simulink model "Tethered_Wind_Tunnel_Test"  (R2023a)
settings: Solver=VariableStepAuto  StartTime=0.0  StopTime=10.0  RelTol=1e-3
values from neighbouring files (symbols this model uses):
  b = 0.490    (= 0.49)    [Cascaded_PI_Step.m]    (also in Cascaded_PI_Zero_Ref.m; Gain_Scheduled_PI_Step.m; Gain_Scheduled_PI_Zero_Ref.m; Inner_Loop_Relay_Feedback.m)
  Bc = 0    [Tethered_Wind_Tunnel.m]
  c = 0.0885    [Tethered_Wind_Tunnel.m]
  Clbc = 1    [Tethered_Wind_Tunnel.m]
  Clda = 0.65    [Cascaded_PI_Step.m]    (also in Cascaded_PI_Zero_Ref.m; Gain_Scheduled_PI_Step.m; Gain_Scheduled_PI_Zero_Ref.m; Inner_Loop_Relay_Feedback.m)
  Cldr = -0.005    [Tethered_Wind_Tunnel.m]
  Clo = 1.108    [Cascaded_PI_Step.m]    (also in Cascaded_PI_Zero_Ref.m; Gain_Scheduled_PI_Step.m; Gain_Scheduled_PI_Zero_Ref.m; Inner_Loop_Relay_Feedback.m)
  Clp = -1.5    [Cascaded_PI_Step.m]    (also in Cascaded_PI_Zero_Ref.m = -11.5; Gain_Scheduled_PI_Step.m = -11.5; Gain_Scheduled_PI_Zero_Ref.m = -11.5; Inner_Loop_Relay_Feedback.m = -11.5)
  Clr = -15.4    [Tethered_Wind_Tunnel.m]
  Cma = -1.26    [Tethered_Wind_Tunnel.m]
  Cmde = 1.34    [Tethered_Wind_Tunnel.m]
  Cmo = 1    [Tethered_Wind_Tunnel.m]
  Cmq = -20.8    [Tethered_Wind_Tunnel.m]
  Cnbc = 1    [Tethered_Wind_Tunnel.m]
  Cnda = -0.065    [Tethered_Wind_Tunnel.m]
  Cndr = 0.005    [Tethered_Wind_Tunnel.m]
  Cno = 1.108    [Tethered_Wind_Tunnel.m]
  Cnp = -12    [Tethered_Wind_Tunnel.m]
  Cnr = -15    [Tethered_Wind_Tunnel.m]
  Gamma1 = (Ixz*(Ix-Iy-Iz))/Gamma0    (= 17.8020633247)    [Tethered_Wind_Tunnel.m]
  Gamma2 = (Iz*(Iz-Iy)+(Ixz^2))/Gamma0    (= -16.6988378289)    [Tethered_Wind_Tunnel.m]
  Gamma5 = (Iz-Ix)/Iy    (= 0.315753887762)    [Tethered_Wind_Tunnel.m]
  Gamma6 = Ixz/Gamma0    (= -13.0686120428)    [Tethered_Wind_Tunnel.m]
  Gamma7 = ((Ix-Iy)*Ix+Ixz^2)/Gamma0    (= -12.4708347919)    [Tethered_Wind_Tunnel.m]
  Iy = 1.0353    [Tethered_Wind_Tunnel.m]
  Kc2 = 7.67    [Cascaded_PI_Step.m]    (also in Cascaded_PI_Zero_Ref.m; Gain_Scheduled_PI_Step.m; Gain_Scheduled_PI_Zero_Ref.m; Tethered_Wind_Tunnel.m)
  Kc3 = 4.5    [Tethered_Wind_Tunnel.m]
  Kc4 = 0.87    [Tethered_Wind_Tunnel.m]
  Kc5 = 0.55    [Tethered_Wind_Tunnel.m]
  phi_des = 30    [Cascaded_PI_Step.m]    (also in Cascaded_PI_Zero_Ref.m = 0; Gain_Scheduled_PI_Step.m; Gain_Scheduled_PI_Zero_Ref.m = 0; Outer_Loop_Relay_Feedback.m = 20)
  r_des = 1    [Tethered_Wind_Tunnel.m]
  rho = 1.204    [Cascaded_PI_Step.m]    (also in Cascaded_PI_Zero_Ref.m; Gain_Scheduled_PI_Step.m; Gain_Scheduled_PI_Zero_Ref.m; Inner_Loop_Relay_Feedback.m)
  S = 0.44    [Cascaded_PI_Step.m]    (also in Cascaded_PI_Zero_Ref.m; Gain_Scheduled_PI_Step.m; Gain_Scheduled_PI_Zero_Ref.m; Inner_Loop_Relay_Feedback.m)
  tau2 = 24.12    [Cascaded_PI_Step.m]    (also in Cascaded_PI_Zero_Ref.m; Gain_Scheduled_PI_Step.m; Gain_Scheduled_PI_Zero_Ref.m; Tethered_Wind_Tunnel.m)
  tau3 = 20.12    [Tethered_Wind_Tunnel.m]
  tau4 = 0.10    (= 0.1)    [Tethered_Wind_Tunnel.m]
  tau5 = 1.25    [Tethered_Wind_Tunnel.m]
  theta_des = 7    [Tethered_Wind_Tunnel.m]
  Va = 15    [Cascaded_PI_Step.m]    (also in Cascaded_PI_Zero_Ref.m; Gain_Scheduled_PI_Step.m; Gain_Scheduled_PI_Zero_Ref.m; Inner_Loop_Relay_Feedback.m)
libraries: slpidlib x5
settings Model: Creator=brend  LastModifiedBy=brend

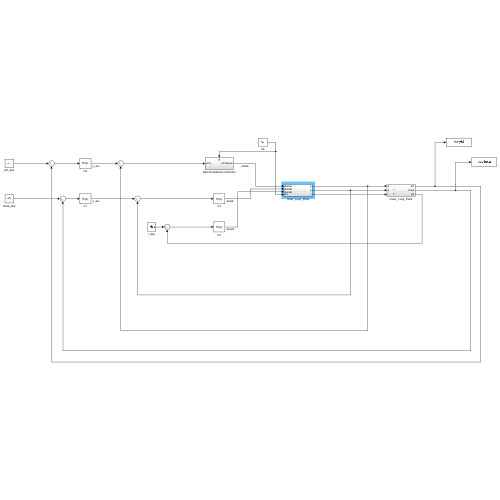
[thumbnail: Simulink's stored preview of the top-level diagram]
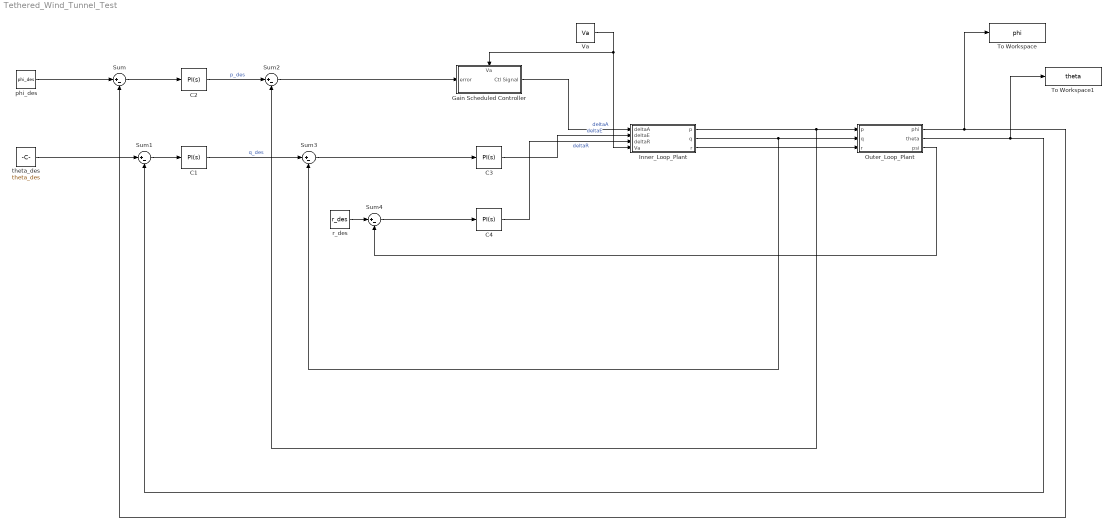
== system Tethered_Wind_Tunnel_Test ==
  C1 : slpidlib/PID Controller  Controller=PI  Form=Parallel  TimeDomain=Continuous-time  UseExternalTs=off  SampleTime=-1  IntegratorMethod=Forward Euler  FilterMethod=Forward Euler  ControllerParametersSource=internal  P=Kc3  I=tau3  UseKiTs=off  D=0  N=100  UseFilter=on  TunerSelectOption=Transfer Function Based (PID Tuner App)  InitialConditionSource=internal  InitialConditionForIntegrator=0  InitialConditionForFilter=0  DifferentiatorICPrevScaledInput=0  ExternalReset=none  TrackingMode=off  Kt=1  LimitOutput=off  SatLimitsSource=internal  UpperSaturationLimit=inf  LowerSaturationLimit=-inf  LinearizeAsGain=on  AntiWindupMode=none  Kb=1  LimitIntegrator=off  UpperIntegratorSaturationLimit=inf  LowerIntegratorSaturationLimit=-inf  POutMin=[]  POutMax=[]  IOutMin=[]  IOutMax=[]  DOutMin=[]  DOutMax=[]  NOutMin=[]  NOutMax=[]  SumOutMin=[]  SumOutMax=[]  SaturationOutMin=[]  SaturationOutMax=[]  PParamMin=[]  PParamMax=[]  IParamMin=[]  IParamMax=[]  DParamMin=[]  DParamMax=[]  NParamMin=[]  NParamMax=[]  KbParamMin=[]  KbParamMax=[]  KtParamMin=[]  KtParamMax=[]  KbOutMin=[]  KbOutMax=[]  KtOutMin=[]  KtOutMax=[]  IntegratorOutMin=[]  IntegratorOutMax=[]  FilterOutMin=[]  FilterOutMax=[]  SumI1OutMin=[]  SumI1OutMax=[]  SumI2OutMin=[]  SumI2OutMax=[]  SumI3OutMin=[]  SumI3OutMax=[]  SumI4OutMin=[]  SumI4OutMax=[]  SumDOutMin=[]  SumDOutMax=[]  DifferentiatorOutMin=[]  DifferentiatorOutMax=[]  FilterDiffOutCoefMin=[]  FilterDiffOutCoefMax=[]  ReciprocalOutMin=[]  ReciprocalOutMax=[]  SumDenOutMin=[]  SumDenOutMax=[]  SumNumOutMin=[]  SumNumOutMax=[]  DivideOutMin=[]  DivideOutMax=[]  UdiffTsProdOutMin=[]  UdiffTsProdOutMax=[]  NTsProdOutMin=[]  NTsProdOutMax=[]  UintegralTsProdOutMin=[]  UintegralTsProdOutMax=[]  UngainTsProdOutMin=[]  UngainTsProdOutMax=[]  ClampingZeroOutDataTypeStr=Inherit: Inherit via back propagation  ClampingZeroOutMin=[]  ClampingZeroOutMax=[]  FilterDenConstantOutDataTypeStr=Inherit: Inherit via back propagation  FilterDenConstantOutMin=[]  FilterDenConstantOutMax=[]  PCopyOutDataTypeStr=Inherit: Inherit via back propagation  PCopyOutMin=[]  PCopyOutMax=[]  NCopyOutDataTypeStr=Inherit: Inherit via back propagation  NCopyOutMin=[]  NCopyOutMax=[]  IntegratorContinuousStateAttributes=''  IntegratorStateMustResolveToSignalObject=off  IntegratorRTWStateStorageClass=Auto  FilterContinuousStateAttributes=''  FilterStateMustResolveToSignalObject=off  FilterRTWStateStorageClass=Auto  ParallelPVariant=InternalParameters  IdealPVariant=Disabled  IVariant=InternalParameters  DVariant=Disabled  IntegratorVariant=Continuous  SatVariant=Disabled  AWVariant=Passthrough  PCopyVariant=Disabled  TRVariant=Disabled  FdbkBlocksVariant=Forward  IdealPFdbkVariant=Disabled  SatFdbkVariant=Disabled  DerivativeFilterVariant=Disabled  NVariant=Disabled  NCopyVariant=Disabled_SignalSpec  FilterICVariant=Disabled  IntegratorICVariant=InternalICs  ExternalResetVariant=Disabled  TRSumVariant=Passthrough  SumFdbkVariant=Disabled  SumVariant=Sum_PI  TsampFilterVariant=InternalTs  TsampNgainVariant=Passthrough  TsampIntegralVariant=Disabled_SignalSpec  ExternalSaturationOutDataTypeStr=Inherit: Same as second input
  C2 : slpidlib/PID Controller  Controller=PI  Form=Parallel  TimeDomain=Continuous-time  UseExternalTs=off  SampleTime=-1  IntegratorMethod=Forward Euler  FilterMethod=Forward Euler  ControllerParametersSource=internal  P=Kc2  I=tau2  UseKiTs=off  D=0  N=100  UseFilter=on  TunerSelectOption=Transfer Function Based (PID Tuner App)  InitialConditionSource=internal  InitialConditionForIntegrator=0  InitialConditionForFilter=0  DifferentiatorICPrevScaledInput=0  ExternalReset=none  TrackingMode=off  Kt=1  LimitOutput=off  SatLimitsSource=internal  UpperSaturationLimit=inf  LowerSaturationLimit=-inf  LinearizeAsGain=on  AntiWindupMode=none  Kb=1  LimitIntegrator=off  UpperIntegratorSaturationLimit=inf  LowerIntegratorSaturationLimit=-inf  POutMin=[]  POutMax=[]  IOutMin=[]  IOutMax=[]  DOutMin=[]  DOutMax=[]  NOutMin=[]  NOutMax=[]  SumOutMin=[]  SumOutMax=[]  SaturationOutMin=[]  SaturationOutMax=[]  PParamMin=[]  PParamMax=[]  IParamMin=[]  IParamMax=[]  DParamMin=[]  DParamMax=[]  NParamMin=[]  NParamMax=[]  KbParamMin=[]  KbParamMax=[]  KtParamMin=[]  KtParamMax=[]  KbOutMin=[]  KbOutMax=[]  KtOutMin=[]  KtOutMax=[]  IntegratorOutMin=[]  IntegratorOutMax=[]  FilterOutMin=[]  FilterOutMax=[]  SumI1OutMin=[]  SumI1OutMax=[]  SumI2OutMin=[]  SumI2OutMax=[]  SumI3OutMin=[]  SumI3OutMax=[]  SumI4OutMin=[]  SumI4OutMax=[]  SumDOutMin=[]  SumDOutMax=[]  DifferentiatorOutMin=[]  DifferentiatorOutMax=[]  FilterDiffOutCoefMin=[]  FilterDiffOutCoefMax=[]  ReciprocalOutMin=[]  ReciprocalOutMax=[]  SumDenOutMin=[]  SumDenOutMax=[]  SumNumOutMin=[]  SumNumOutMax=[]  DivideOutMin=[]  DivideOutMax=[]  UdiffTsProdOutMin=[]  UdiffTsProdOutMax=[]  NTsProdOutMin=[]  NTsProdOutMax=[]  UintegralTsProdOutMin=[]  UintegralTsProdOutMax=[]  UngainTsProdOutMin=[]  UngainTsProdOutMax=[]  ClampingZeroOutDataTypeStr=Inherit: Inherit via back propagation  ClampingZeroOutMin=[]  ClampingZeroOutMax=[]  FilterDenConstantOutDataTypeStr=Inherit: Inherit via back propagation  FilterDenConstantOutMin=[]  FilterDenConstantOutMax=[]  PCopyOutDataTypeStr=Inherit: Inherit via back propagation  PCopyOutMin=[]  PCopyOutMax=[]  NCopyOutDataTypeStr=Inherit: Inherit via back propagation  NCopyOutMin=[]  NCopyOutMax=[]  IntegratorContinuousStateAttributes=''  IntegratorStateMustResolveToSignalObject=off  IntegratorRTWStateStorageClass=Auto  FilterContinuousStateAttributes=''  FilterStateMustResolveToSignalObject=off  FilterRTWStateStorageClass=Auto  ParallelPVariant=InternalParameters  IdealPVariant=Disabled  IVariant=InternalParameters  DVariant=Disabled  IntegratorVariant=Continuous  SatVariant=Disabled  AWVariant=Passthrough  PCopyVariant=Disabled  TRVariant=Disabled  FdbkBlocksVariant=Forward  IdealPFdbkVariant=Disabled  SatFdbkVariant=Disabled  DerivativeFilterVariant=Disabled  NVariant=Disabled  NCopyVariant=Disabled_SignalSpec  FilterICVariant=Disabled  IntegratorICVariant=InternalICs  ExternalResetVariant=Disabled  TRSumVariant=Passthrough  SumFdbkVariant=Disabled  SumVariant=Sum_PI  TsampFilterVariant=InternalTs  TsampNgainVariant=Passthrough  TsampIntegralVariant=Disabled_SignalSpec  ExternalSaturationOutDataTypeStr=Inherit: Same as second input
  C3 : slpidlib/PID Controller  Controller=PI  Form=Parallel  TimeDomain=Continuous-time  UseExternalTs=off  SampleTime=-1  IntegratorMethod=Forward Euler  FilterMethod=Forward Euler  ControllerParametersSource=internal  P=Kc4  I=tau4  UseKiTs=off  D=0  N=100  UseFilter=on  TunerSelectOption=Transfer Function Based (PID Tuner App)  InitialConditionSource=internal  InitialConditionForIntegrator=0  InitialConditionForFilter=0  DifferentiatorICPrevScaledInput=0  ExternalReset=none  TrackingMode=off  Kt=1  LimitOutput=off  SatLimitsSource=internal  UpperSaturationLimit=inf  LowerSaturationLimit=-inf  LinearizeAsGain=on  AntiWindupMode=none  Kb=1  LimitIntegrator=off  UpperIntegratorSaturationLimit=inf  LowerIntegratorSaturationLimit=-inf  POutMin=[]  POutMax=[]  IOutMin=[]  IOutMax=[]  DOutMin=[]  DOutMax=[]  NOutMin=[]  NOutMax=[]  SumOutMin=[]  SumOutMax=[]  SaturationOutMin=[]  SaturationOutMax=[]  PParamMin=[]  PParamMax=[]  IParamMin=[]  IParamMax=[]  DParamMin=[]  DParamMax=[]  NParamMin=[]  NParamMax=[]  KbParamMin=[]  KbParamMax=[]  KtParamMin=[]  KtParamMax=[]  KbOutMin=[]  KbOutMax=[]  KtOutMin=[]  KtOutMax=[]  IntegratorOutMin=[]  IntegratorOutMax=[]  FilterOutMin=[]  FilterOutMax=[]  SumI1OutMin=[]  SumI1OutMax=[]  SumI2OutMin=[]  SumI2OutMax=[]  SumI3OutMin=[]  SumI3OutMax=[]  SumI4OutMin=[]  SumI4OutMax=[]  SumDOutMin=[]  SumDOutMax=[]  DifferentiatorOutMin=[]  DifferentiatorOutMax=[]  FilterDiffOutCoefMin=[]  FilterDiffOutCoefMax=[]  ReciprocalOutMin=[]  ReciprocalOutMax=[]  SumDenOutMin=[]  SumDenOutMax=[]  SumNumOutMin=[]  SumNumOutMax=[]  DivideOutMin=[]  DivideOutMax=[]  UdiffTsProdOutMin=[]  UdiffTsProdOutMax=[]  NTsProdOutMin=[]  NTsProdOutMax=[]  UintegralTsProdOutMin=[]  UintegralTsProdOutMax=[]  UngainTsProdOutMin=[]  UngainTsProdOutMax=[]  ClampingZeroOutDataTypeStr=Inherit: Inherit via back propagation  ClampingZeroOutMin=[]  ClampingZeroOutMax=[]  FilterDenConstantOutDataTypeStr=Inherit: Inherit via back propagation  FilterDenConstantOutMin=[]  FilterDenConstantOutMax=[]  PCopyOutDataTypeStr=Inherit: Inherit via back propagation  PCopyOutMin=[]  PCopyOutMax=[]  NCopyOutDataTypeStr=Inherit: Inherit via back propagation  NCopyOutMin=[]  NCopyOutMax=[]  IntegratorContinuousStateAttributes=''  IntegratorStateMustResolveToSignalObject=off  IntegratorRTWStateStorageClass=Auto  FilterContinuousStateAttributes=''  FilterStateMustResolveToSignalObject=off  FilterRTWStateStorageClass=Auto  ParallelPVariant=InternalParameters  IdealPVariant=Disabled  IVariant=InternalParameters  DVariant=Disabled  IntegratorVariant=Continuous  SatVariant=Disabled  AWVariant=Passthrough  PCopyVariant=Disabled  TRVariant=Disabled  FdbkBlocksVariant=Forward  IdealPFdbkVariant=Disabled  SatFdbkVariant=Disabled  DerivativeFilterVariant=Disabled  NVariant=Disabled  NCopyVariant=Disabled_SignalSpec  FilterICVariant=Disabled  IntegratorICVariant=InternalICs  ExternalResetVariant=Disabled  TRSumVariant=Passthrough  SumFdbkVariant=Disabled  SumVariant=Sum_PI  TsampFilterVariant=InternalTs  TsampNgainVariant=Passthrough  TsampIntegralVariant=Disabled_SignalSpec  ExternalSaturationOutDataTypeStr=Inherit: Same as second input
  C4 : slpidlib/PID Controller  Controller=PI  Form=Parallel  TimeDomain=Continuous-time  UseExternalTs=off  SampleTime=-1  IntegratorMethod=Forward Euler  FilterMethod=Forward Euler  ControllerParametersSource=internal  P=Kc5  I=tau5  UseKiTs=off  D=0  N=100  UseFilter=on  TunerSelectOption=Transfer Function Based (PID Tuner App)  InitialConditionSource=internal  InitialConditionForIntegrator=0  InitialConditionForFilter=0  DifferentiatorICPrevScaledInput=0  ExternalReset=none  TrackingMode=off  Kt=1  LimitOutput=off  SatLimitsSource=internal  UpperSaturationLimit=inf  LowerSaturationLimit=-inf  LinearizeAsGain=on  AntiWindupMode=none  Kb=1  LimitIntegrator=off  UpperIntegratorSaturationLimit=inf  LowerIntegratorSaturationLimit=-inf  POutMin=[]  POutMax=[]  IOutMin=[]  IOutMax=[]  DOutMin=[]  DOutMax=[]  NOutMin=[]  NOutMax=[]  SumOutMin=[]  SumOutMax=[]  SaturationOutMin=[]  SaturationOutMax=[]  PParamMin=[]  PParamMax=[]  IParamMin=[]  IParamMax=[]  DParamMin=[]  DParamMax=[]  NParamMin=[]  NParamMax=[]  KbParamMin=[]  KbParamMax=[]  KtParamMin=[]  KtParamMax=[]  KbOutMin=[]  KbOutMax=[]  KtOutMin=[]  KtOutMax=[]  IntegratorOutMin=[]  IntegratorOutMax=[]  FilterOutMin=[]  FilterOutMax=[]  SumI1OutMin=[]  SumI1OutMax=[]  SumI2OutMin=[]  SumI2OutMax=[]  SumI3OutMin=[]  SumI3OutMax=[]  SumI4OutMin=[]  SumI4OutMax=[]  SumDOutMin=[]  SumDOutMax=[]  DifferentiatorOutMin=[]  DifferentiatorOutMax=[]  FilterDiffOutCoefMin=[]  FilterDiffOutCoefMax=[]  ReciprocalOutMin=[]  ReciprocalOutMax=[]  SumDenOutMin=[]  SumDenOutMax=[]  SumNumOutMin=[]  SumNumOutMax=[]  DivideOutMin=[]  DivideOutMax=[]  UdiffTsProdOutMin=[]  UdiffTsProdOutMax=[]  NTsProdOutMin=[]  NTsProdOutMax=[]  UintegralTsProdOutMin=[]  UintegralTsProdOutMax=[]  UngainTsProdOutMin=[]  UngainTsProdOutMax=[]  ClampingZeroOutDataTypeStr=Inherit: Inherit via back propagation  ClampingZeroOutMin=[]  ClampingZeroOutMax=[]  FilterDenConstantOutDataTypeStr=Inherit: Inherit via back propagation  FilterDenConstantOutMin=[]  FilterDenConstantOutMax=[]  PCopyOutDataTypeStr=Inherit: Inherit via back propagation  PCopyOutMin=[]  PCopyOutMax=[]  NCopyOutDataTypeStr=Inherit: Inherit via back propagation  NCopyOutMin=[]  NCopyOutMax=[]  IntegratorContinuousStateAttributes=''  IntegratorStateMustResolveToSignalObject=off  IntegratorRTWStateStorageClass=Auto  FilterContinuousStateAttributes=''  FilterStateMustResolveToSignalObject=off  FilterRTWStateStorageClass=Auto  ParallelPVariant=InternalParameters  IdealPVariant=Disabled  IVariant=InternalParameters  DVariant=Disabled  IntegratorVariant=Continuous  SatVariant=Disabled  AWVariant=Passthrough  PCopyVariant=Disabled  TRVariant=Disabled  FdbkBlocksVariant=Forward  IdealPFdbkVariant=Disabled  SatFdbkVariant=Disabled  DerivativeFilterVariant=Disabled  NVariant=Disabled  NCopyVariant=Disabled_SignalSpec  FilterICVariant=Disabled  IntegratorICVariant=InternalICs  ExternalResetVariant=Disabled  TRSumVariant=Passthrough  SumFdbkVariant=Disabled  SumVariant=Sum_PI  TsampFilterVariant=InternalTs  TsampNgainVariant=Passthrough  TsampIntegralVariant=Disabled_SignalSpec  ExternalSaturationOutDataTypeStr=Inherit: Same as second input
  Gain Scheduled Controller : Subsystem
      settings: PortSchema="{\"entries\":[{\"content\":{\"sides\":[{\"content\":{\"connectorIds\":[\"In1\"]},\"type\":\"ConnectorPlacement.EquallySpacedRectSide\",\"uuid\":\"2e087caa-f72d-4490-8964-36fbcf7716d7\"},{\"content\":{\"connectorIds\":[\"Out1\"],\"side\":\"RIGHT\"},\"type\":\"ConnectorPlacement.EquallySpacedRectSide\",\"uuid\":\"b0dafe2c-6d7a-42e1-bf72-883c5565d2ef\"},{\"content\":{\"connectorIds\":[\"In2\"],\"side\":\"TOP\"},\"type\":\"ConnectorPlacement.EquallySpacedRectSide\",\"uuid\":\"4416cd10-6726-4ba3-b71a-642a6449d506\"}]},\"type\":\"ConnectorPlacement.EquallySpacedConnector\",\"uuid\":\"4db1e7fb-938c-4dd4-ad91-0eb120ffb4c4\"}],\"packageUris\":[\"http://schema.mathworks.com/mf0/Connector/R2020b\"],\"version\":\"1.0\"}"
  Inner_Loop_Plant : Subsystem
  Outer_Loop_Plant : Subsystem
  Sum{,1..4} (5 alike) : Sum  Inputs=|+-
  To Workspace : ToWorkspace  VariableName=phi  SaveFormat=Timeseries  SampleTime=-1
  To Workspace1 : ToWorkspace  VariableName=theta  SaveFormat=Timeseries  SampleTime=-1
  Va : Constant  Value=Va
  phi_des : Constant  Value=phi_des
  r_des : Constant  Value=r_des
  theta_des : Constant  Value=theta_des
  wires:
  phi_des/1 -> Sum/1
  theta_des/1 -> Sum1/1
  Outer_Loop_Plant/3(psi) -> Sum4/2
  Outer_Loop_Plant/1(phi) -> To Workspace/1, Sum/2
  Inner_Loop_Plant/1(p) -> Outer_Loop_Plant/1(p), Sum2/2
  Inner_Loop_Plant/2(q) -> Sum3/2, Outer_Loop_Plant/2(q)
  Inner_Loop_Plant/3(r) -> Outer_Loop_Plant/3(r)
  Va/1 -> Gain Scheduled Controller/2(Va), Inner_Loop_Plant/4(Va)
  r_des/1 -> Sum4/1
  Sum2/1 -> Gain Scheduled Controller/1(error)
  C2/1 -> Sum2/1  "p_des"
  Sum/1 -> C2/1
  Sum1/1 -> C1/1
  C1/1 -> Sum3/1  "q_des"
  Sum3/1 -> C3/1
  Sum4/1 -> C4/1
  Gain Scheduled Controller/1(Ctl Signal) -> Inner_Loop_Plant/1(deltaA)  "deltaA"
  C3/1 -> Inner_Loop_Plant/2(deltaE)  "deltaE"
  C4/1 -> Inner_Loop_Plant/3(deltaR)  "deltaR"
  Outer_Loop_Plant/2(theta) -> To Workspace1/1, Sum1/2

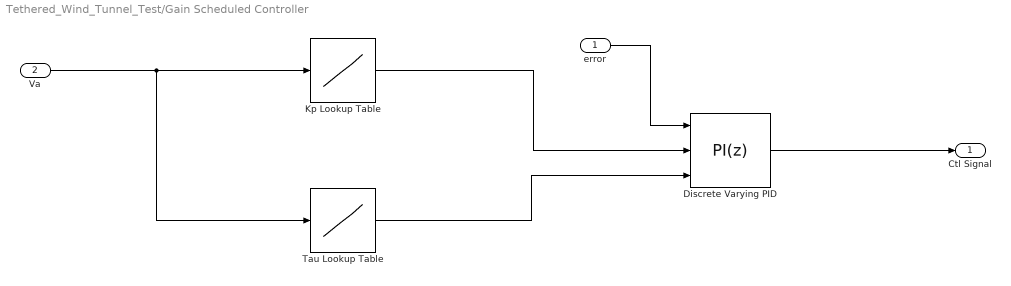
== system Tethered_Wind_Tunnel_Test/Gain Scheduled Controller ==
  error : Inport
  Va : Inport  Port=2
  Discrete Varying PID : slpidlib/PID Controller  Controller=PI  Form=Parallel  TimeDomain=Discrete-time  UseExternalTs=off  SampleTime=-1  IntegratorMethod=Forward Euler  FilterMethod=Forward Euler  ControllerParametersSource=external  P=1  I=1  UseKiTs=off  D=0  N=100  UseFilter=on  TunerSelectOption=Transfer Function Based (PID Tuner App)  InitialConditionSource=internal  InitialConditionForIntegrator=0  InitialConditionForFilter=0  DifferentiatorICPrevScaledInput=0  ExternalReset=none  TrackingMode=off  Kt=1  LimitOutput=off  SatLimitsSource=internal  UpperSaturationLimit=inf  LowerSaturationLimit=-inf  LinearizeAsGain=on  AntiWindupMode=none  Kb=1  LimitIntegrator=off  UpperIntegratorSaturationLimit=inf  LowerIntegratorSaturationLimit=-inf  POutMin=[]  POutMax=[]  IOutMin=[]  IOutMax=[]  DOutMin=[]  DOutMax=[]  NOutMin=[]  NOutMax=[]  SumOutMin=[]  SumOutMax=[]  SaturationOutMin=[]  SaturationOutMax=[]  PParamMin=[]  PParamMax=[]  IParamMin=[]  IParamMax=[]  DParamMin=[]  DParamMax=[]  NParamMin=[]  NParamMax=[]  KbParamMin=[]  KbParamMax=[]  KtParamMin=[]  KtParamMax=[]  KbOutMin=[]  KbOutMax=[]  KtOutMin=[]  KtOutMax=[]  IntegratorOutMin=[]  IntegratorOutMax=[]  FilterOutMin=[]  FilterOutMax=[]  SumI1OutMin=[]  SumI1OutMax=[]  SumI2OutMin=[]  SumI2OutMax=[]  SumI3OutMin=[]  SumI3OutMax=[]  SumI4OutMin=[]  SumI4OutMax=[]  SumDOutMin=[]  SumDOutMax=[]  DifferentiatorOutMin=[]  DifferentiatorOutMax=[]  FilterDiffOutCoefMin=[]  FilterDiffOutCoefMax=[]  ReciprocalOutMin=[]  ReciprocalOutMax=[]  SumDenOutMin=[]  SumDenOutMax=[]  SumNumOutMin=[]  SumNumOutMax=[]  DivideOutMin=[]  DivideOutMax=[]  UdiffTsProdOutMin=[]  UdiffTsProdOutMax=[]  NTsProdOutMin=[]  NTsProdOutMax=[]  UintegralTsProdOutMin=[]  UintegralTsProdOutMax=[]  UngainTsProdOutMin=[]  UngainTsProdOutMax=[]  ClampingZeroOutDataTypeStr=Inherit: Inherit via back propagation  ClampingZeroOutMin=[]  ClampingZeroOutMax=[]  FilterDenConstantOutDataTypeStr=Inherit: Inherit via back propagation  FilterDenConstantOutMin=[]  FilterDenConstantOutMax=[]  PCopyOutDataTypeStr=Inherit: Inherit via back propagation  PCopyOutMin=[]  PCopyOutMax=[]  NCopyOutDataTypeStr=Inherit: Inherit via back propagation  NCopyOutMin=[]  NCopyOutMax=[]  IntegratorContinuousStateAttributes=''  IntegratorStateMustResolveToSignalObject=off  IntegratorRTWStateStorageClass=Auto  FilterContinuousStateAttributes=''  FilterStateMustResolveToSignalObject=off  FilterRTWStateStorageClass=Auto  ParallelPVariant=ExternalParameters  IdealPVariant=Disabled  IVariant=ExternalParameters  DVariant=Disabled  IntegratorVariant=Discrete  SatVariant=Disabled  AWVariant=Passthrough  PCopyVariant=Disabled  TRVariant=Disabled  FdbkBlocksVariant=Forward  IdealPFdbkVariant=Disabled  SatFdbkVariant=Disabled  DerivativeFilterVariant=Disabled  NVariant=Disabled  NCopyVariant=Disabled_SignalSpec  FilterICVariant=Disabled  IntegratorICVariant=InternalICs  ExternalResetVariant=Disabled  TRSumVariant=Passthrough  SumFdbkVariant=Disabled  SumVariant=Sum_PI  TsampFilterVariant=InternalTs  TsampNgainVariant=Passthrough  TsampIntegralVariant=Disabled_SignalSpec  ExternalSaturationOutDataTypeStr=Inherit: Same as second input
      settings: LibrarySourceBlock=cstblocks/Linear Parameter Varying/Discrete Varying PID
  Kp Lookup Table : Lookup_n-D  NumberOfTableDimensions=1  BreakpointsForDimension1=[-5:5]  Table=tanh([-5:5])  InternalRulePriority=Speed  RndMeth=Simplest
  Tau Lookup Table : Lookup_n-D  NumberOfTableDimensions=1  BreakpointsForDimension1=[-5:5]  Table=tanh([-5:5])  InternalRulePriority=Speed  RndMeth=Simplest
  Ctl Signal : Outport
  wires:
  Va/1 -> Tau Lookup Table/1, Kp Lookup Table/1
  Kp Lookup Table/1 -> Discrete Varying PID/2
  Tau Lookup Table/1 -> Discrete Varying PID/3
  error/1 -> Discrete Varying PID/1
  Discrete Varying PID/1 -> Ctl Signal/1

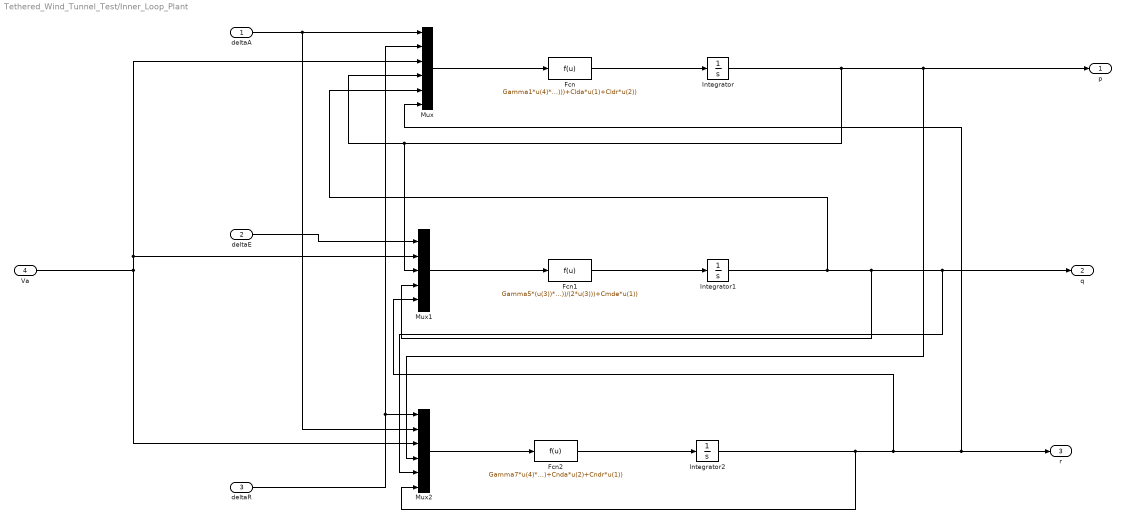
== system Tethered_Wind_Tunnel_Test/Inner_Loop_Plant ==
  deltaA : Inport
  deltaE : Inport  Port=2
  deltaR : Inport  Port=3
  Va : Inport  Port=4
  Fcn : Fcn  Expr=Gamma1*u(4)*u(5)-Gamma2*u(5)*u(6)+0.5*rho*((u(3))^2)*S*b*(Clo + Clbc*Bc + Clp*((b*u(4))/(2*u(3)))+Clr*((b*u(6))/(2*u(3)))+Clda*u(1)+Cldr*u(2))
  Fcn1 : Fcn  Expr=Gamma5*(u(3))*(u(5)) - Gamma6*((u(3))^2-(u(5))^2) + ((rho*(u(2))^2*S*c)/(2*Iy))*(Cmo + Cma + Cmq*((c*u(4))/(2*u(3)))+Cmde*u(1))
  Fcn2 : Fcn  Expr=Gamma7*u(4)*u(5)-Gamma1*u(5)*u(6)+0.5*rho*(u(3)^2)*S*b*(Cno + Cnbc*Bc + Cnp*((b*u(4))/(2*u(3)))+Cnr*((b*u(6))/(2*u(3)))+Cnda*u(2)+Cndr*u(1))
  Integrator : Integrator  UpperSaturationLimit=100  LowerSaturationLimit=-100
  Integrator1 : Integrator
  Integrator2 : Integrator
  Mux : Mux  Inputs=6
  Mux1 : Mux  Inputs=5
  Mux2 : Mux  Inputs=6
  p : Outport
  q : Outport  Port=2
  r : Outport  Port=3
  wires:
  deltaA/1 -> Mux2/2, Mux/1
  deltaR/1 -> Mux2/1, Mux/2
  Va/1 -> Mux2/3, Mux1/2, Mux/3
  Mux/1 -> Fcn/1
  Fcn/1 -> Integrator/1
  Integrator/1 -> Mux1/3, Mux/4, Mux2/4, p/1
  deltaE/1 -> Mux1/1
  Mux1/1 -> Fcn1/1
  Fcn1/1 -> Integrator1/1
  Integrator1/1 -> Mux/5, Mux1/4, Mux2/5, q/1
  Integrator2/1 -> Mux2/6, Mux1/5, Mux/6, r/1
  Fcn2/1 -> Integrator2/1
  Mux2/1 -> Fcn2/1

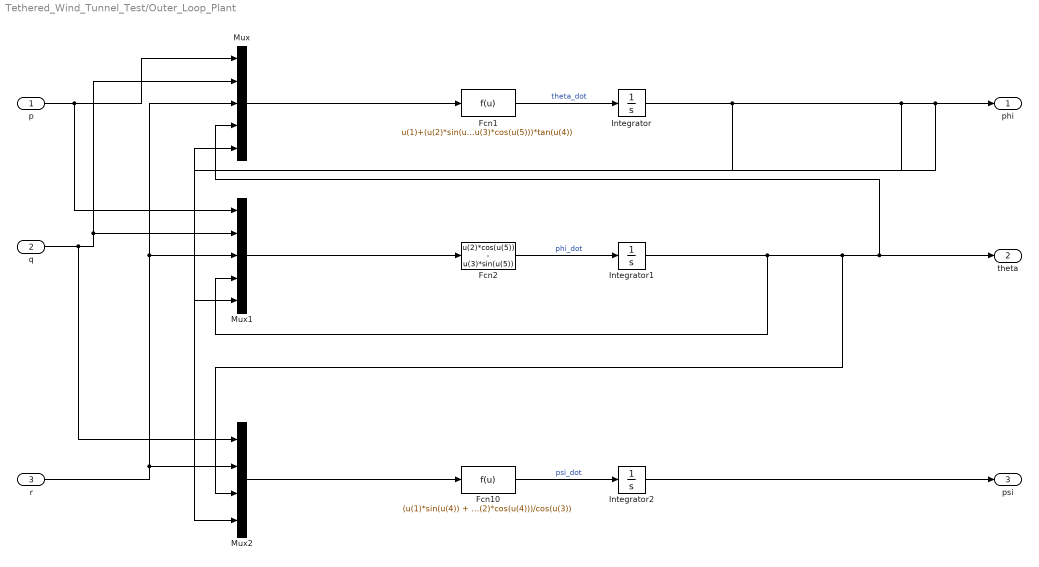
== system Tethered_Wind_Tunnel_Test/Outer_Loop_Plant ==
  p : Inport
  q : Inport  Port=2
  r : Inport  Port=3
  Fcn1 : Fcn  Expr=u(1)+(u(2)*sin(u(5)) + u(3)*cos(u(5)))*tan(u(4))
  Fcn10 : Fcn  Expr=(u(1)*sin(u(4)) + u(2)*cos(u(4)))/cos(u(3))
  Fcn2 : Fcn  Expr=u(2)*cos(u(5)) - u(3)*sin(u(5))
  Integrator : Integrator
  Integrator1 : Integrator
  Integrator2 : Integrator
  Mux : Mux  Inputs=5
  Mux1 : Mux  Inputs=5
  Mux2 : Mux
  phi : Outport
  theta : Outport  Port=2
  psi : Outport  Port=3
  wires:
  p/1 -> Mux1/1, Mux/1
  q/1 -> Mux2/1, Mux1/2, Mux/2
  r/1 -> Mux1/3, Mux/3, Mux2/2
  Mux/1 -> Fcn1/1
  Fcn1/1 -> Integrator/1  "theta_dot"
  Integrator/1 -> Mux/5, Mux1/5, Mux2/4, phi/1
  Fcn2/1 -> Integrator1/1  "phi_dot"
  Integrator1/1 -> Mux1/4, Mux2/3, theta/1, Mux/4
  Fcn10/1 -> Integrator2/1  "psi_dot"
  Integrator2/1 -> psi/1
  Mux2/1 -> Fcn10/1
  Mux1/1 -> Fcn2/1
